simulink model "Control_PID_Tanque01"  (R2013a)
settings: Solver=ode45  StartTime=0.0  StopTime=1000  RelTol=1e-3
InitFcn:
  | load('Kp.mat')
  | load('Kd.mat')
  | load('Ki.mat')
undefined symbols (not defined in the file or in its folder): sigbuilder_block
undefined symbols (not defined in the file): Kd, Ki, Kp
libraries: simulink x1
settings Model: Creator=Cristhian Ivan  LastModifiedBy=Cristhian Ivan

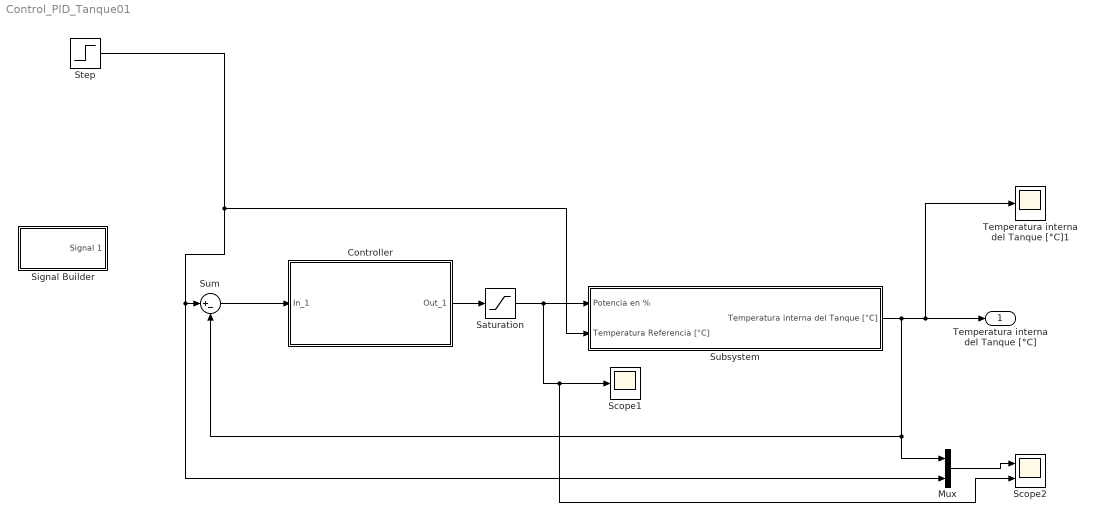
== system Control_PID_Tanque01 ==
  Controller : Subsystem  mask(PID Controller){P=Kp, I=Ki, D=Kd}
      mask prompts: P "Proportional:"; I "Integral"; D "Derivative:"
      mask help: Enter expressions for proportional, integral, and derivative terms.
      mask Help: This block implements a PID controller where paramaters are entered for the Proportional, Integral and Derivative terms.
      mask Display: disp('PID')
  Mux : Mux  Inputs=2
  Saturation : Saturate  UpperLimit=100  LowerLimit=-100  ZeroCross=off
  Scope1 : Scope
      settings: SaveName=ScopeData2
  Scope2 : Scope  NumInputPorts=2
      settings: YMin=-5~-5  YMax=5~5
  Signal Builder : Subsystem  Tag=STV Subsys  LoadFcn=sigbuilder_block('load');  StartFcn=sigbuilder_block('start');  StopFcn=sigbuilder_block('stop');  ClipboardFcn=sigbuilder_block('clipboard');  mask(Sigbuilder block){}
      mask help: Simulink:masks:SigbuilderBlock_MD
      mask init:
      | if ~strcmp(get_param(bdroot(gcbh),'SimulationStatus'),'stopped') tuvar = sigbuilder_block('maskInit'); end
      settings: CopyFcn=sigbuilder_block('copy');  DeleteFcn=sigbuilder_block('delete');  ModelCloseFcn=sigbuilder_block('modelClose');  PreSaveFcn=sigbuilder_block('preSave');  PauseFcn=sigbuilder_block('pause');  ContinueFcn=sigbuilder_block('continue');  NameChangeFcn=sigbuilder_block('namechange');  OpenFcn=sigbuilder_block('open',[437.25 118.5 550.5 394.5 ]);  CloseFcn=sigbuilder_block('close');
      mask Display: plot(0, 0, 100, 100,[2, 2, 32, 32, 2], [68, 8, 8, 68, 68],[32, 2], [38, 38], [32, 19, 2],[53, 60, 44], [32, 17, 17, 2],[16, 16, 31, 31]);txt = getActiveGroup(gcbh);text(2, 100, txt,'verticalAlignment', 'top');
  Step : Step  Time=0  After=42  SampleTime=0
  Subsystem : Subsystem
  Sum : Sum  Inputs=|+-
  Temperatura interna del Tanque [°C]1 : Scope
      settings: TimeRange=10  YMin=20  YMax=45  SaveName=TransResp
  Temperatura interna del Tanque [°C] : Outport
  wires:
  Subsystem/1(Temperatura interna del Tanque [°C]) -> Temperatura interna del Tanque [°C]1/1, Temperatura interna del Tanque [°C]/1, Mux/1, Sum/2
  Sum/1 -> Controller/1(In_1)
  Mux/1 -> Scope2/1
  Step/1 -> Subsystem/2(Temperatura Referencia [°C]), Mux/2, Sum/1
  Controller/1(Out_1) -> Saturation/1
  Saturation/1 -> Scope2/2, Scope1/1, Subsystem/1(Potencia en %)

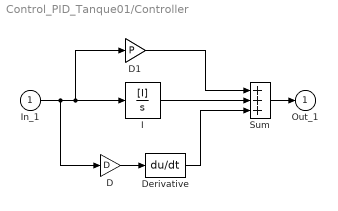
== system Control_PID_Tanque01/Controller ==
  In_1 : Inport
  D : Gain  Gain=D  SaturateOnIntegerOverflow=on  OutDataTypeStr=Inherit: Same as input  ParamDataTypeStr=Inherit: Same as input
  D1 : Gain  Gain=P  SaturateOnIntegerOverflow=on  OutDataTypeStr=Inherit: Same as input  ParamDataTypeStr=Inherit: Same as input
  Derivative : Derivative
  I : TransferFcn  Numerator=[I]  Denominator=[1 0]
  Sum : Sum  Inputs=+++  SaturateOnIntegerOverflow=on  InputSameDT=on  OutDataTypeStr=Inherit: Same as first input
  Out_1 : Outport  InitialOutput=0
  wires:
  In_1/1 -> D1/1, I/1, D/1
  Sum/1 -> Out_1/1
  D/1 -> Derivative/1
  Derivative/1 -> Sum/3
  I/1 -> Sum/2
  D1/1 -> Sum/1

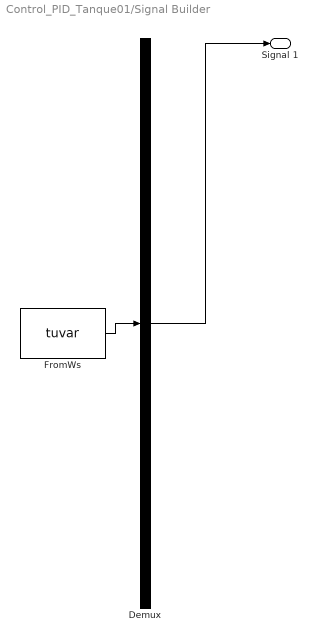
== system Control_PID_Tanque01/Signal Builder ==
  Demux : Demux  Tag=STV Demux  Outputs=1
  FromWs : FromWorkspace  Tag=STV FromWs  VariableName=tuvar  SampleTime=0
      SigBuilderData=|
      | common.afterFinalStr = 'Extrapolate'
      | common.sampleTime = 0
      | dataSet.timeRange = [0 1000]
      | dataSet.name = 'Group 1'
      | sbobj.Groups.Name = 'Group 1'
      | sbobj.Groups.Signals.Name = 'Signal 1'
      | sbobj.Groups.Signals.XData = [0 44 44 400 400 738 738 1000]
      | sbobj.Groups.Signals.YData = [35 35 40.05 40.05 30.4 30.4 38.05 38.05]
      | sbobj.Groups.TimeRange = [0 1000]
  Signal 1 : Outport  Tag=STV Outport
  wires:
  Demux/1 -> Signal 1/1
  FromWs/1 -> Demux/1

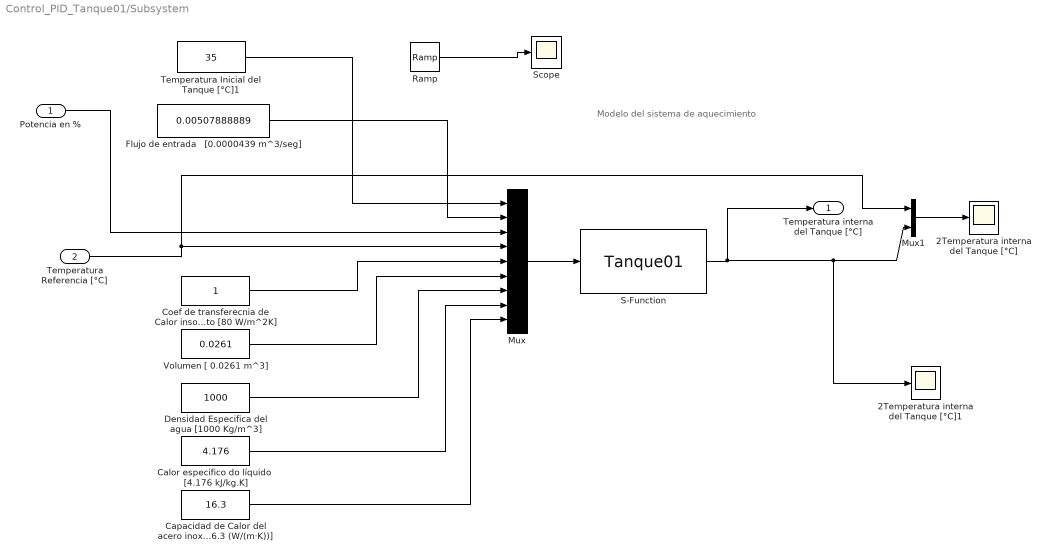
== system Control_PID_Tanque01/Subsystem ==
  note: Modelo del sistema de aquecimiento
  Potencia en % : Inport
  Temperatura Referencia [°C] : Inport  Port=2
  2Temperatura interna del Tanque [°C] : Scope
      settings: TimeRange=10  YMin=20  YMax=45
  2Temperatura interna del Tanque [°C]1 : Scope
      settings: TimeRange=10  YMin=20  YMax=45  SaveName=RespSimulada
  Calor especifico do líquido  [4.176 kJ/kg.K] : Constant  Value=4.176
  Capacidad de Calor del acero inox [16.3 (W/(m·K))] : Constant  Value=16.3
  Coef de transferecnia de Calor insolamiento [80 W/m^2K] : Constant
  Densidad Especifica del agua [1000 Kg/m^3] : Constant  Value=1000
  "Flujo de entrada   [0.0000439 m^3/seg] " : Constant  Value=0.00507888889
  Mux : Mux  Inputs=9
  Mux1 : Mux  Inputs=2
  Ramp : simulink/Sources/Ramp  slope=0.01  start=26  X0=26
  S-Function : S-Function  FunctionName=Tanque01  EnableBusSupport=off
  Scope : Scope
      settings: SaveName=ScopeData3
  Temperatura Inicial del Tanque [°C]1 : Constant  Value=35
  Volumen [ 0.0261 m^3] : Constant  Value=0.0261
  Temperatura interna del Tanque [°C] : Outport
  wires:
  Mux1/1 -> 2Temperatura interna del Tanque [°C]/1
  Capacidad de Calor del acero inox [16.3 (W/(m·K))]/1 -> Mux/9
  Volumen [ 0.0261 m^3]/1 -> Mux/6
  "Flujo de entrada   [0.0000439 m^3/seg] "/1 -> Mux/2
  Densidad Especifica del agua [1000 Kg/m^3]/1 -> Mux/7
  Mux/1 -> S-Function/1
  Coef de transferecnia de Calor insolamiento [80 W/m^2K]/1 -> Mux/5
  S-Function/1 -> Temperatura interna del Tanque [°C]/1, 2Temperatura interna del Tanque [°C]1/1, Mux1/2
  Calor especifico do líquido  [4.176 kJ/kg.K]/1 -> Mux/8
  Temperatura Referencia [°C]/1 -> Mux1/1, Mux/4
  Potencia en %/1 -> Mux/3
  Ramp/1 -> Scope/1
  Temperatura Inicial del Tanque [°C]1/1 -> Mux/1
